simulink model "Lab5_Task1_2_3"  (R2014b)
settings: Solver=ode45  StartTime=0.0  StopTime=2  RelTol=1e-3
settings Model: Creator=Eduardo  LastModifiedBy=Eduardo Montilva

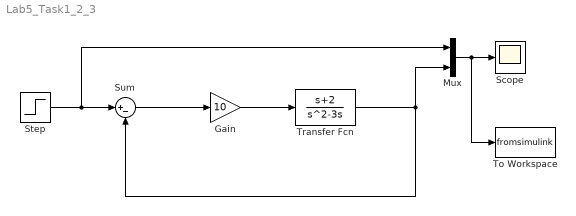
== system Lab5_Task1_2_3 ==
  Gain : Gain  Gain=10
  Mux : Mux  Inputs=2
  Scope : Scope
  Step : Step  Time=0  SampleTime=0
  Sum : Sum  Inputs=|+-
  To Workspace : ToWorkspace  VariableName=fromsimulink  SaveFormat=Timeseries  SampleTime=-1
  Transfer Fcn : TransferFcn  Numerator=[1 2]  Denominator=[1 -3 0]
  wires:
  Step/1 -> Mux/1, Sum/1
  Transfer Fcn/1 -> Mux/2, Sum/2
  Sum/1 -> Gain/1
  Gain/1 -> Transfer Fcn/1
  Mux/1 -> To Workspace/1, Scope/1
